simulink model "ExampleDynamicMesh"  (R2024a)
settings: Solver=FixedStepAuto  StartTime=0.0  StopTime=inf  FixedStep=0.02  RelTol=1e-3  EnableMultiTasking=on
undefined symbols (not defined in the file): color, invRadiusPow4, meshID, pointLightID, position, quadraticFalloff, quaternion, shouldBeDeleted, updateMesh, visible
libraries: PRISMA x10, GenericTarget x1
settings Model: Creator=damerius  LastModifiedBy=Scythe
settings SolverCC: ConcurrentTasks=on  AlgebraicLoopSolver=TrustRegion  PositivePriorityOrder=on
settings DataIOCC: SaveOutput=off  SignalLogging=off  DSMLogging=off  SaveTime=off  ReturnWorkspaceOutputs=off
settings OptimizationCC: DefaultParameterBehavior=Inlined  ReuseModelBlockBuffer=off  ZeroExternalMemoryAtStartup=off  ZeroInternalMemoryAtStartup=off  SimCompilerOptimization=on
settings DebuggingCC: UnconnectedInputMsg=warning  UnconnectedOutputMsg=warning  UnconnectedLineMsg=warning
settings HardwareCC: ProdBitPerLong=64  ProdHWDeviceType=Intel->x86-64 (Linux 64)
settings ModelReferenceCC: EnableRefExpFcnMdlSchedulingChecks=on
settings SFSimCC: SimParseCustomCode=off  SimGenImportedTypeDefs=on  SimTargetLang=C++
settings RTWCC: GenCodeOnly=on  PackageGeneratedCodeAndArtifacts=on  PackageName=PackNGo  RTWVerbose=off  BuildConfiguration=Faster Runs  TargetLang=C++  GPUComputeCapability=3.5  DLArmComputeVersion=19.05
settings CodeAppCC: ForceParamTrailComments=on  MaxIdLength=95  MATLABSourceComments=on  UseSimReservedNames=on
settings GRTTargetCC: TargetLangStandard=C++11 (ISO)  GenerateFullHeader=off  MatFileLogging=off  CodeInterfacePackaging=C++ class

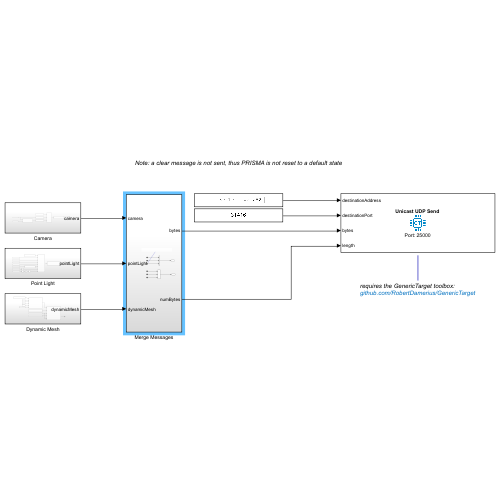
[thumbnail: Simulink's stored preview of the top-level diagram]
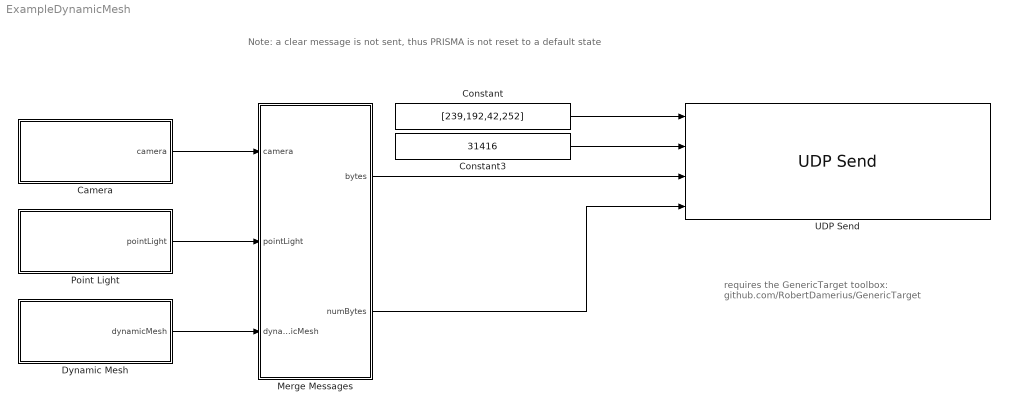
== system ExampleDynamicMesh ==
  note: Note: a clear message is not sent, thus PRISMA is not reset to a default state
  note: requires the GenericTarget toolbox:
      | github.com/RobertDamerius/GenericTarget
  Camera : Subsystem
  Constant : Constant  Value=[239,192,42,252]  OutDataTypeStr=uint8
  Constant3 : Constant  Value=31416  OutDataTypeStr=uint16
  Dynamic Mesh : Subsystem
  Merge Messages : Subsystem
  Point Light : Subsystem
  UDP Send : GenericTarget/Interface/UDP Send  showDetails=off  interfacePort=25000  interfaceIP=[0,0,0,0]  deviceName=''  prioritySocket=6  allowBroadcast=off  SampleTime=-1
      settings: SourceProductName=Generic Target
  wires:
  Constant3/1 -> UDP Send/2
  Camera/1(camera) -> Merge Messages/1(camera)
  Dynamic Mesh/1(dynamicMesh) -> Merge Messages/3(dynamicMesh)
  Merge Messages/1(bytes) -> UDP Send/3
  Merge Messages/2(numBytes) -> UDP Send/4
  Point Light/1(pointLight) -> Merge Messages/2(pointLight)
  Constant/1 -> UDP Send/1

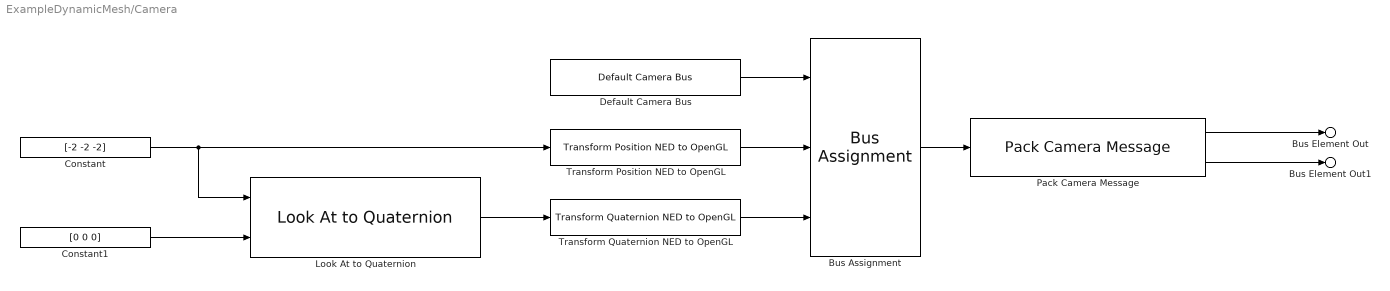
== system ExampleDynamicMesh/Camera ==
  Bus Assignment : BusAssignment  AssignedSignals=position,quaternion
  Constant : Constant  Value=[-2 -2 -2]
  Constant1 : Constant  Value=[0 0 0]
  Default Camera Bus : PRISMA/Default Camera Bus
      settings: SourceProductName=PRISMA
  Look At to Quaternion : PRISMA/Transformation/Look At to Quaternion
      settings: SourceProductName=PRISMA
  Pack Camera Message : PRISMA/Pack Camera Message
      settings: SourceProductName=PRISMA
  Transform Position NED to OpenGL : PRISMA/Transformation/Transform Position NED to OpenGL
      settings: SourceProductName=PRISMA
  Transform Quaternion NED to OpenGL : PRISMA/Transformation/Transform Quaternion NED to OpenGL
      settings: SourceProductName=PRISMA
  Bus Element Out : Outport  PortName=camera  Element=bytes
  Bus Element Out1 : Outport  PortName=camera  Element=numBytes
  wires:
  Default Camera Bus/1 -> Bus Assignment/1
  Bus Assignment/1 -> Pack Camera Message/1
  Transform Position NED to OpenGL/1 -> Bus Assignment/2
  Transform Quaternion NED to OpenGL/1 -> Bus Assignment/3
  Look At to Quaternion/1 -> Transform Quaternion NED to OpenGL/1
  Constant/1 -> Look At to Quaternion/1, Transform Position NED to OpenGL/1
  Constant1/1 -> Look At to Quaternion/2
  Pack Camera Message/1 -> Bus Element Out/1
  Pack Camera Message/2 -> Bus Element Out1/1

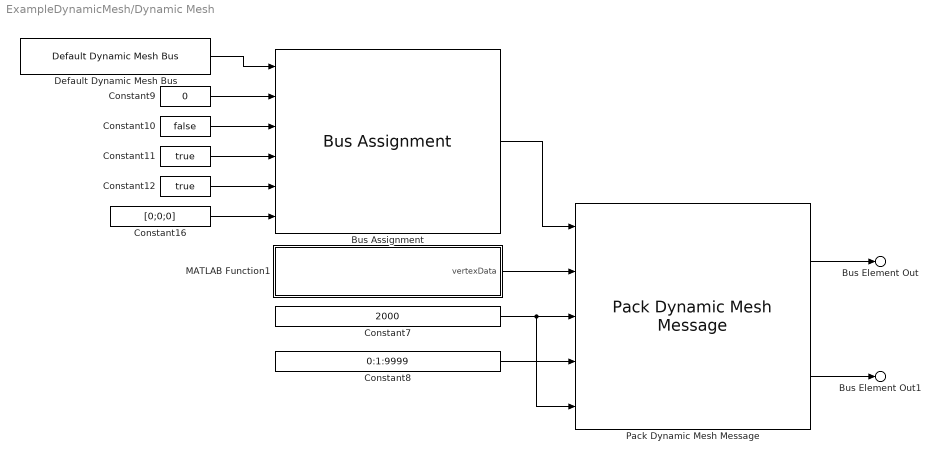
== system ExampleDynamicMesh/Dynamic Mesh ==
  Bus Assignment : BusAssignment  AssignedSignals=meshID,shouldBeDeleted,updateMesh,visible,position
  Constant10 : Constant  Value=false  OutDataTypeStr=boolean
  Constant11 : Constant  Value=true  OutDataTypeStr=boolean
  Constant12 : Constant  Value=true  OutDataTypeStr=boolean
  Constant16 : Constant  Value=[0;0;0]  OutDataTypeStr=double
  Constant7 : Constant  Value=2000
  Constant8 : Constant  Value=0:1:9999
  Constant9 : Constant  Value=0  OutDataTypeStr=uint32
  Default Dynamic Mesh Bus : PRISMA/Default Dynamic Mesh Bus
      settings: SourceProductName=PRISMA
  MATLAB Function1 : MATLAB Function  TreatAsAtomicUnit=on
  Pack Dynamic Mesh Message : PRISMA/Pack Dynamic Mesh Message
      settings: SourceProductName=PRISMA
  Bus Element Out : Outport  PortName=dynamicMesh  Element=bytes
  Bus Element Out1 : Outport  PortName=dynamicMesh  Element=numBytes
  wires:
  Constant10/1 -> Bus Assignment/3
  Constant16/1 -> Bus Assignment/6
  Constant12/1 -> Bus Assignment/5
  Bus Assignment/1 -> Pack Dynamic Mesh Message/1
  Constant7/1 -> Pack Dynamic Mesh Message/3, Pack Dynamic Mesh Message/5
  Default Dynamic Mesh Bus/1 -> Bus Assignment/1
  Constant8/1 -> Pack Dynamic Mesh Message/4
  MATLAB Function1/1(vertexData) -> Pack Dynamic Mesh Message/2
  Constant9/1 -> Bus Assignment/2
  Constant11/1 -> Bus Assignment/4
  Pack Dynamic Mesh Message/1 -> Bus Element Out/1
  Pack Dynamic Mesh Message/2 -> Bus Element Out1/1

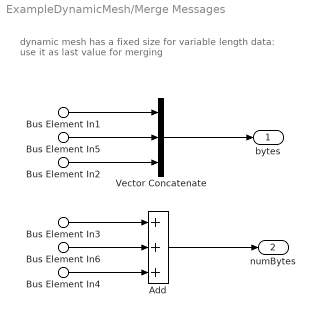
== system ExampleDynamicMesh/Merge Messages ==
  note: dynamic mesh has a fixed size for variable length data:
      | use it as last value for merging
  Bus Element In1 : Inport  PortName=camera  Element=bytes
  Bus Element In3 : Inport  PortName=camera  Element=numBytes
  Bus Element In5 : Inport  Port=2  PortName=pointLight  Element=bytes
  Bus Element In6 : Inport  Port=2  PortName=pointLight  Element=numBytes
  Bus Element In2 : Inport  Port=3  PortName=dynamicMesh  Element=bytes
  Bus Element In4 : Inport  Port=3  PortName=dynamicMesh  Element=numBytes
  Add : Sum  Inputs=+++
  Vector Concatenate : Concatenate  NumInputs=3
  bytes : Outport
  numBytes : Outport  Port=2
  wires:
  Bus Element In1/1 -> Vector Concatenate/1
  Bus Element In2/1 -> Vector Concatenate/3
  Bus Element In3/1 -> Add/1
  Bus Element In4/1 -> Add/3
  Vector Concatenate/1 -> bytes/1
  Add/1 -> numBytes/1
  Bus Element In5/1 -> Vector Concatenate/2
  Bus Element In6/1 -> Add/2

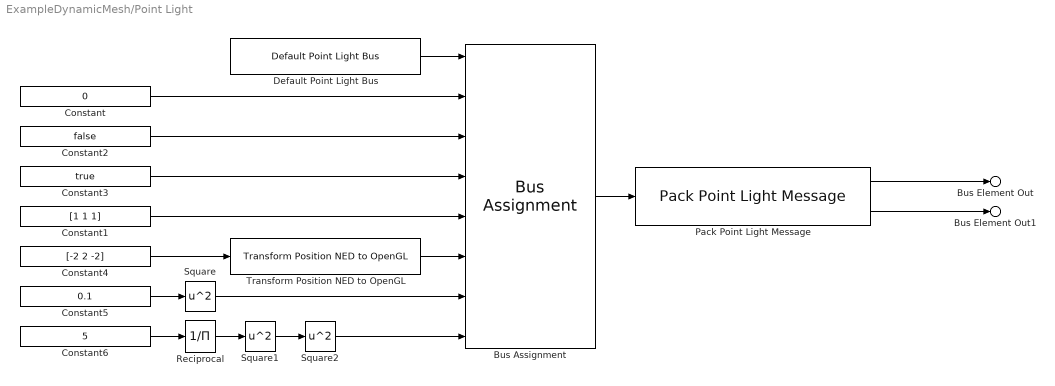
== system ExampleDynamicMesh/Point Light ==
  Bus Assignment : BusAssignment  AssignedSignals=pointLightID,shouldBeDeleted,visible,color,position,quadraticFalloff,invRadiusPow4
  Constant : Constant  Value=0  OutDataTypeStr=uint32
  Constant1 : Constant  Value=[1 1 1]
  Constant2 : Constant  Value=false  OutDataTypeStr=boolean
  Constant3 : Constant  Value=true  OutDataTypeStr=boolean
  Constant4 : Constant  Value=[-2 2 -2]
  Constant5 : Constant  Value=0.1
  Constant6 : Constant  Value=5
  Default Point Light Bus : PRISMA/Default Point Light Bus
      settings: SourceProductName=PRISMA
  Pack Point Light Message : PRISMA/Pack Point Light Message
      settings: SourceProductName=PRISMA
  Reciprocal : Product  Inputs=/
  Square : Math  Operator=square
  Square1 : Math  Operator=square
  Square2 : Math  Operator=square
  Transform Position NED to OpenGL : PRISMA/Transformation/Transform Position NED to OpenGL
      settings: SourceProductName=PRISMA
  Bus Element Out : Outport  PortName=pointLight  Element=bytes
  Bus Element Out1 : Outport  PortName=pointLight  Element=numBytes
  wires:
  Pack Point Light Message/2 -> Bus Element Out1/1
  Pack Point Light Message/1 -> Bus Element Out/1
  Bus Assignment/1 -> Pack Point Light Message/1
  Default Point Light Bus/1 -> Bus Assignment/1
  Constant/1 -> Bus Assignment/2
  Constant2/1 -> Bus Assignment/3
  Constant3/1 -> Bus Assignment/4
  Constant1/1 -> Bus Assignment/5
  Transform Position NED to OpenGL/1 -> Bus Assignment/6
  Constant4/1 -> Transform Position NED to OpenGL/1
  Constant5/1 -> Square/1
  Square/1 -> Bus Assignment/7
  Reciprocal/1 -> Square1/1
  Square1/1 -> Square2/1
  Square2/1 -> Bus Assignment/8
  Constant6/1 -> Reciprocal/1

== matlab function ExampleDynamicMesh/Dynamic Mesh/MATLAB Function1 ==
  data: vertexData output
function vertexData = RandomVertices()
    vertexData = [rand(3,2000)*2.0 - 1.0; rand(3,2000)]; % position and color
end
